simulink library "VLSGains"  (R2022b)
settings: Solver=VariableStepAuto  StartTime=0.0  StopTime=10.0  RelTol=1e-3
values from neighbouring files (symbols this model uses):
  VLSGainsConfig = struct('sample_rate_in_hertz', sample_rate_in_hertz,                              'frame_size', frame_size,                              'rgain_SILENT_GAIN', rgain_SILENT_GAIN,                              'granularity', internal_granularity,                              'numGains', numGains)    [VLSGainsInit.m]
  VLSGainsTune = load(VLSGainsTuneFileName)    [VLSGainsInit.m]
undefined symbols (not defined in the file or in its folder): Row
libraries: TuneVar x36, TOP x18, FeaturePath x2
(part 2 of 2)

== matlab function VLSGains/VLS Gains Pax/Fade Tuning/Forward Downmix Threshold/Trivial Translation ==
  data: TOP output; ForwardDownmixThreshold input
  events: trigger input FUNCTION_CALL_EVENT
function TOP  = fcn(ForwardDownmixThreshold)
%#codegen
% Checks if the parameter satisfies dimensionality requirements
if(numel(ForwardDownmixThreshold.Value) ~= 1)
   TranslateError('The parameter ''medusa_forward_downmix_threshold'' must be single dimensional.'); 
end

% Checks if the parameter value follows bound requirements
if((ForwardDownmixThreshold.Value < 0) || (ForwardDownmixThreshold.Value > 1))
   TranslateError('The value of ''medusa_forward_downmix_threshold'' must be between 0 and 1.'); 
end

TOP = ForwardDownmixThreshold.Value;

end

== matlab function VLSGains/VLS Gains Pax/Fade Tuning/Foward Downmix Max/Trivial Translation ==
  data: TOP output; ForwardDownmixMax input
  events: trigger input FUNCTION_CALL_EVENT
function TOP  = fcn(ForwardDownmixMax)
%#codegen
% Checks if the parameter satisfies dimensionality requirements
if(numel(ForwardDownmixMax.Value) ~= 1)
   TranslateError('The parameter ''medusa_forward_downmix_max'' must be single dimensional.'); 
end

% Checks if the parameter value follows bound requirements
if((ForwardDownmixMax.Value < 0) || (ForwardDownmixMax.Value > 1))
   TranslateError('The value of ''medusa_forward_downmix_max'' must be between 0 and 1.'); 
end

TOP = ForwardDownmixMax.Value;

end

== matlab function VLSGains/VLS Gains Pax/Gain Computation/Fader Downmix/MATLAB Function ==
  data: forwardGain input; downmix output; forwardDownmixThreshold input; forwardDownmixMax input; backwardGain input; backwardDownmixThreshold input; backwardDownmixMax input
function downmix = fcn(forwardGain, forwardDownmixThreshold, forwardDownmixMax,...
    backwardGain, backwardDownmixThreshold, backwardDownmixMax)

if (forwardGain >= backwardGain)
    downmix = (1 - min(backwardGain, forwardDownmixThreshold) / max(forwardDownmixThreshold, single(eps)))...
        * forwardDownmixMax;
else
    downmix = (1 - min(forwardGain, backwardDownmixThreshold) / max(backwardDownmixThreshold, single(eps)))...
        * backwardDownmixMax;
end

== matlab function VLSGains/VLS Gains Pax/Gain Computation/Ramper/check sequence ==
  data: done output; VLSPax_currentGain data_store_memory; VLSPax_targetGain data_store_memory
  events: trigger input FUNCTION_CALL_EVENT
function done = GetCompletedSequence
% #codegen

    global VLSPax_currentGain;
    global VLSPax_targetGain;

    % Assume the work is complete until proven otherwise
    done = true;

    for i=1:numel(VLSPax_targetGain)
       if (VLSPax_targetGain(i) ~= VLSPax_currentGain(i))
           done = false; % just proved otherwise
           break;
       end
    end

end

== matlab function VLSGains/VLS Gains Pax/Gain Computation/Ramper/control ==
  data target_gains_linear settings: description=This vector signal must provide a linear target gain for every ramper.
  data: target_gains_linear input; rampRate input; rampTime input; configStruct parameter; VLSPax_Freeze data_store_memory; VLSPax_frameCount data_store_memory; VLSPax_rampCoeff data_store_memory; VLSPax_targetGain data_store_memory; VLSPax_currentGain data_store_memory
  events: trigger input FUNCTION_CALL_EVENT
function control(target_gains_linear, rampRate, rampTime, configStruct)
%#codegen

    global VLSPax_Freeze;
    global VLSPax_frameCount;
    global VLSPax_rampCoeff;
    global VLSPax_targetGain;
    global VLSPax_currentGain;  

    dim_rgain = size(VLSPax_currentGain);
    rgain_SILENT_GAIN_mat = (configStruct.rgain_SILENT_GAIN)*ones(dim_rgain);

    % Step 1: FREEZE the gain ramper so that we can perform calculations based
    % on the current gain value.
    VLSPax_Freeze(1) = true; % freeze the gain

    % Step 2: Nudge the gain values a bit if they are sitting at zero.
    % When this control set goes live, ensure that the current gain will move.
    % If current gain is zero, replace with a value very close to zero. What we
    % really want is a value which is on the edge of perception - not too small
    % or large. If the value is too small, we'll waste some of our ramp time
    % in perceived silence. If the value is too large, the audio will lurch
    % into perceptability at the start of the ramp.
    currentgain = max(VLSPax_currentGain, rgain_SILENT_GAIN_mat);
    targetGain  = max(target_gains_linear, rgain_SILENT_GAIN_mat);
    
    % Step 3a: If a ramp time in milliseconds is provided, ignore the ramp
    % rate in dB/sec (if also provided), otherwise calculate a new ramp time
    % that matches the slope.
    rampTime_ms = single(rampTime)*ones(dim_rgain);
    
    if(~rampTime)
        currentGain_db = 20*log10(currentgain);
        targetGain_db = 20*log10(targetGain);
        diff = abs(currentGain_db - targetGain_db);
        rampTime_ms = diff / single(rampRate) * 1000;
    end
    
    % Step 3b: QUANTIZE the desired ramp time to our FrameSize. Also retrieve 
    % the whole number of frames required to best match requested ramp time.
    % Ensure that at least one frame is used. The frame size will therefore
    % determine the steepest ramp (i.e. within one frame you can go anywhere).
    quantum_ms = 1000 * (configStruct.frame_size) / (configStruct.sample_rate_in_hertz);
    numFrames = rampTime_ms / quantum_ms;
    numFrames = max (1, round(numFrames));

    % In order to have the desired ramp time, the slope must vary dependent
    % on the gain differencebetween target and current value.
    % Ramper's coefficient is therefore calculated as follows:
    %
    %   TargetGain = CurrentGain *( RampCoef ^ (Fs*RampTime_ms/1000) )
    %
    % therefore...
    %
    %                     log(TargetGain/CurrentGain)
    %   log(RampCoef) = ------------------------------
    %                        Fs*(RampTime_ms/1000)
    %
    factor = log( targetGain ./ currentgain );
    RampCoef = exp(factor ./ numFrames);

    % Output control signals
    VLSPax_frameCount  = int32(numFrames);
    VLSPax_rampCoeff   = single(RampCoef);
    VLSPax_targetGain  = target_gains_linear;
    VLSPax_currentGain = currentgain;

    % unfreeze the gain
    VLSPax_Freeze(1) = false;

end

== matlab function VLSGains/VLS Gains Pax/Gain Computation/Ramper/process ==
  data: VLSPax_Freeze data_store_memory; VLSPax_currentGain data_store_memory; VLSPax_targetGain data_store_memory; VLSPax_frameCount data_store_memory; VLSPax_rampCoeff data_store_memory
function process
%#codegen

    global VLSPax_Freeze;
    global VLSPax_currentGain;
    global VLSPax_targetGain;
    global VLSPax_frameCount;
    global VLSPax_rampCoeff;
    
    for i = 1:numel(VLSPax_currentGain)
        if (VLSPax_Freeze(1) == false)
            if (VLSPax_frameCount(i) == 0)
                % The ramp is finished. Stop ramping and SNAP to the target
                VLSPax_currentGain(i) = VLSPax_targetGain(i);
            else
                % The ramp is *NOT* frozen or done: gain is moving
                VLSPax_currentGain(i) = VLSPax_currentGain(i)*VLSPax_rampCoeff(i);
                VLSPax_frameCount(i) = VLSPax_frameCount(i) - 1;
            end
        end
    end
    
end

== matlab function VLSGains/VLS Gains Drv/Gain Computation/Fader Downmix/MATLAB Function ==
  data: forwardGain input; downmix output; forwardDownmixThreshold input; forwardDownmixMax input; backwardGain input; backwardDownmixThreshold input; backwardDownmixMax input
function downmix = fcn(forwardGain, forwardDownmixThreshold, forwardDownmixMax,...
    backwardGain, backwardDownmixThreshold, backwardDownmixMax)

if (forwardGain >= backwardGain)
    downmix = (1 - min(backwardGain, forwardDownmixThreshold) / max(forwardDownmixThreshold, single(eps)))...
        * forwardDownmixMax;
else
    downmix = (1 - min(forwardGain, backwardDownmixThreshold) / max(backwardDownmixThreshold, single(eps)))...
        * backwardDownmixMax;
end

== matlab function VLSGains/VLS Gains Drv/Gain Computation/Surround Level Control/Initialization and RMDL ==
  data: minGain input; detentGain input; maxGain input; interpolation_method input; surr_level input; configStruct parameter; VLSDrv_currentGain data_store_memory; VLSDrv_targetGain data_store_memory; VLSDrv_frameCount data_store_memory; VLSDrv_SLCGain data_store_memory
  events: trigger input FUNCTION_CALL_EVENT
function generate_gain(minGain, detentGain, maxGain, interpolation_method, surr_level, configStruct)
% #codegen
    global VLSDrv_currentGain;
    global VLSDrv_targetGain;
    global VLSDrv_SLCGain;
    global VLSDrv_frameCount;

    % Computing the 'surround' part of mixing gains depending on the surround
    % level index; The other part of mixing gain comes from 'fade downmix'
    gain = MedusaPremixGainComputation(minGain, detentGain, maxGain, interpolation_method, surr_level, configStruct);

    % Ramping doesn't take place during RMDL and cold start. Hence, gains
    % are directly pushed to mixing matrix
    VLSDrv_currentGain = gain;
    VLSDrv_targetGain = gain;
    VLSDrv_SLCGain = gain;
    
    % Resetting the frame count to zero to avoid unintentional ramping
    VLSDrv_frameCount = zeros(size(VLSDrv_currentGain), 'int32');
end

== matlab function VLSGains/VLS Gains Pax/Gain Computation/Surround Level Control/Initialization and RMDL ==
  data: minGain input; detentGain input; maxGain input; interpolation_method input; surr_level input; configStruct parameter; VLSPax_currentGain data_store_memory; VLSPax_targetGain data_store_memory; VLSPax_frameCount data_store_memory; VLSPax_SLCGain data_store_memory
  events: trigger input FUNCTION_CALL_EVENT
function generate_gain(minGain, detentGain, maxGain, interpolation_method, surr_level, configStruct)
% #codegen
    global VLSPax_currentGain;
    global VLSPax_targetGain;
    global VLSPax_SLCGain;
    global VLSPax_frameCount;

    % Computing the 'surround' part of mixing gains depending on the surround
    % level index; The other part of mixing gain comes from 'fade downmix'
    gain = MedusaPremixGainComputation(minGain, detentGain, maxGain, interpolation_method, surr_level, configStruct);

    % Ramping doesn't take place during RMDL and cold start. Hence, gains
    % are directly pushed to mixing matrix
    VLSPax_currentGain = gain;
    VLSPax_targetGain = gain;
    VLSPax_SLCGain = gain;
    
    % Resetting the frame count to zero to avoid unintentional ramping
    VLSPax_frameCount = zeros(size(VLSPax_currentGain), 'int32');
end

== matlab function VLSGains/VLS Gains Pax/Gain Computation/Surround Level Control/Target Gain Computation ==
  data: minGain input; detentGain input; maxGain input; interpolation_method input; surr_level input; configStruct parameter; VLSPax_SLCGain data_store_memory
  events: trigger input FUNCTION_CALL_EVENT
function generate_gain(minGain, detentGain, maxGain, interpolation_method, surr_level, configStruct)
% #codegen
    global VLSPax_SLCGain;

    % Computing the 'surround' part of mixing gains depending on the surround
    % level index; The other part of mixing gain comes from 'fade downmix'
    targetGain = MedusaPremixGainComputation(minGain, detentGain, maxGain, interpolation_method, surr_level, configStruct);
    
    VLSPax_SLCGain = targetGain;
end

== matlab function VLSGains/VLS Gains Pax/Generate Ramp Trigger/MATLAB Function ==
  data: SLC_On input; Fade_On input; rampOn output
  events: ramp output FUNCTION_CALL_EVENT
function rampOn = triggerRamp(SLC_On, Fade_On)
%#codegen
rampOn = 0;         % DEBUG parameter

% Trigger ramping if SLC OR Fade is triggered
if(SLC_On || Fade_On)
    rampOn = 1;
    ramp();
end

end

== matlab function VLSGains/VLS Gains Pax/SLC Tuning/Detent Level/Trivial Translation ==
  data: TOP output; detentGain input; configStruct parameter
  events: trigger input FUNCTION_CALL_EVENT
function TOP  = fcn(detentGain, configStruct)
%#codegen

% Checks if the parameter satisfies dimensionality requirements
if(detentGain.Size(1) ~= configStruct.numGains)
    TranslateError('The parameter ''VLS_gains_detent'' must be a %d element vector.', configStruct.numGains);
end

% Checks if the parameter values follow bound requirements
checkValues = (detentGain.Value < 0);    
if(sum(sum(checkValues)))       % Results in 0 if all values in the matrix respect the bound requirements
    TranslateError('The weights in ''VLS_gains_detent'' must be greater than or equal to 0.');
end

TOP = detentGain.Value;

end

== matlab function VLSGains/VLS Gains Pax/SLC Tuning/Interpolation Method/Trivial Translation ==
  data: TOP output; interpolationMethod input
  events: trigger input FUNCTION_CALL_EVENT
function TOP  = fcn(interpolationMethod)
%#codegen
% Checks if the parameter satisfies dimensionality requirements
if(numel(interpolationMethod.Value) ~= 1)
   TranslateError('The parameter ''medusa_surround_db_interpolation'' must be single dimensional.'); 
end

% Checks if the parameter value follows bound requirements
if((interpolationMethod.Value ~= 0) && (interpolationMethod.Value ~= 1))
   TranslateError('The value of ''medusa_surround_db_interpolation'' must be either 0 (for linear interpolation) or 1 (for dB-linear interpolation).'); 
end

TOP = interpolationMethod.Value;

end

== matlab function VLSGains/VLS Gains Pax/SLC Tuning/Max Level/Trivial Translation ==
  data: TOP output; maxGain input; configStruct parameter
  events: trigger input FUNCTION_CALL_EVENT
function TOP  = fcn(maxGain, configStruct)
%#codegen

% Checks if the parameter satisfies dimensionality requirements
if(maxGain.Size(1) ~= configStruct.numGains)
    TranslateError('The parameter ''VLS_gains_max'' must be a %d element vector.', configStruct.numGains);
end

% Checks if the parameter values follow bound requirements
checkValues = (maxGain.Value < 0);
if(sum(sum(checkValues)))          % Results in 0 if all values in the matrix respect the bound requirements
    TranslateError('The weights in ''VLS_gains_max'' must be greater than or equal to 0.');
end

TOP = maxGain.Value;

end

== matlab function VLSGains/VLS Gains Pax/SLC Tuning/Min Level/Trivial Translation ==
  data: TOP output; minGain input; configStruct parameter
  events: trigger input FUNCTION_CALL_EVENT
function TOP  = fcn(minGain, configStruct)
%#codegen

% Checks if the parameter satisfies dimensionality requirements
if(minGain.Size(1) ~= configStruct.numGains)
    TranslateError('The parameter ''VLS_gains_min'' must be a %d element vector.', configStruct.numGains);
end

% Checks if the parameter values follow bound requirements
checkValues = (minGain.Value < 0);
if(sum(sum(checkValues)))          % Results in 0 if all values in the matrix respect the bound requirements
    TranslateError('The weights in ''VLS_gains_min'' must be greater than or equal to 0.');
end

TOP = minGain.Value;

end

== matlab function VLSGains/VLS Gains Drv/Gain Computation/Surround Level Control/Target Gain Computation ==
  data: minGain input; detentGain input; maxGain input; interpolation_method input; surr_level input; configStruct parameter; VLSDrv_SLCGain data_store_memory
  events: trigger input FUNCTION_CALL_EVENT
function generate_gain(minGain, detentGain, maxGain, interpolation_method, surr_level, configStruct)
% #codegen
    global VLSDrv_SLCGain;

    % Computing the 'surround' part of mixing gains depending on the surround
    % level index; The other part of mixing gain comes from 'fade downmix'
    targetGain = MedusaPremixGainComputation(minGain, detentGain, maxGain, interpolation_method, surr_level, configStruct);
    
    VLSDrv_SLCGain = targetGain;
end

== matlab function VLSGains/VLS Gains Drv/SLC Tuning/Detent Level/Trivial Translation ==
  data: TOP output; detentGain input; configStruct parameter
  events: trigger input FUNCTION_CALL_EVENT
function TOP  = fcn(detentGain, configStruct)
%#codegen

% Checks if the parameter satisfies dimensionality requirements
if(detentGain.Size(1) ~= configStruct.numGains)
    TranslateError('The parameter ''VLS_gains_detent'' must be a %d element vector.', configStruct.numGains);
end

% Checks if the parameter values follow bound requirements
checkValues = (detentGain.Value < 0);    
if(sum(sum(checkValues)))       % Results in 0 if all values in the matrix respect the bound requirements
    TranslateError('The weights in ''VLS_gains_detent'' must be greater than or equal to 0.');
end

TOP = detentGain.Value;

end

== matlab function VLSGains/VLS Gains Drv/SLC Tuning/Interpolation Method/Trivial Translation ==
  data: TOP output; interpolationMethod input
  events: trigger input FUNCTION_CALL_EVENT
function TOP  = fcn(interpolationMethod)
%#codegen
% Checks if the parameter satisfies dimensionality requirements
if(numel(interpolationMethod.Value) ~= 1)
   TranslateError('The parameter ''medusa_surround_db_interpolation'' must be single dimensional.'); 
end

% Checks if the parameter value follows bound requirements
if((interpolationMethod.Value ~= 0) && (interpolationMethod.Value ~= 1))
   TranslateError('The value of ''medusa_surround_db_interpolation'' must be either 0 (for linear interpolation) or 1 (for dB-linear interpolation).'); 
end

TOP = interpolationMethod.Value;

end

== matlab function VLSGains/VLS Gains Drv/SLC Tuning/Max Level/Trivial Translation ==
  data: TOP output; maxGain input; configStruct parameter
  events: trigger input FUNCTION_CALL_EVENT
function TOP  = fcn(maxGain, configStruct)
%#codegen

% Checks if the parameter satisfies dimensionality requirements
if(maxGain.Size(1) ~= configStruct.numGains)
    TranslateError('The parameter ''VLS_gains_max'' must be a %d element vector.', configStruct.numGains);
end

% Checks if the parameter values follow bound requirements
checkValues = (maxGain.Value < 0);
if(sum(sum(checkValues)))          % Results in 0 if all values in the matrix respect the bound requirements
    TranslateError('The weights in ''VLS_gains_max'' must be greater than or equal to 0.');
end

TOP = maxGain.Value;

end

== matlab function VLSGains/VLS Gains Drv/SLC Tuning/Min Level/Trivial Translation ==
  data: TOP output; minGain input; configStruct parameter
  events: trigger input FUNCTION_CALL_EVENT
function TOP  = fcn(minGain, configStruct)
%#codegen

% Checks if the parameter satisfies dimensionality requirements
if(minGain.Size(1) ~= configStruct.numGains)
    TranslateError('The parameter ''VLS_gains_min'' must be a %d element vector.', configStruct.numGains);
end

% Checks if the parameter values follow bound requirements
checkValues = (minGain.Value < 0);
if(sum(sum(checkValues)))          % Results in 0 if all values in the matrix respect the bound requirements
    TranslateError('The weights in ''VLS_gains_min'' must be greater than or equal to 0.');
end

TOP = minGain.Value;

end

== matlab function VLSGains/VLS Gains Drv/Gain Computation/Ramper/check sequence ==
  data: done output; VLSDrv_currentGain data_store_memory; VLSDrv_targetGain data_store_memory
  events: trigger input FUNCTION_CALL_EVENT
function done = GetCompletedSequence
% #codegen

    global VLSDrv_currentGain;
    global VLSDrv_targetGain;

    % Assume the work is complete until proven otherwise
    done = true;

    for i=1:numel(VLSDrv_targetGain)
       if (VLSDrv_targetGain(i) ~= VLSDrv_currentGain(i))
           done = false; % just proved otherwise
           break;
       end
    end

end

== matlab function VLSGains/VLS Gains Drv/Gain Computation/Ramper/control ==
  data target_gains_linear settings: description=This vector signal must provide a linear target gain for every ramper.
  data: target_gains_linear input; rampRate input; rampTime input; configStruct parameter; VLSDrv_Freeze data_store_memory; VLSDrv_frameCount data_store_memory; VLSDrv_rampCoeff data_store_memory; VLSDrv_targetGain data_store_memory; VLSDrv_currentGain data_store_memory
  events: trigger input FUNCTION_CALL_EVENT
function control(target_gains_linear, rampRate, rampTime, configStruct)
%#codegen

    global VLSDrv_Freeze;
    global VLSDrv_frameCount;
    global VLSDrv_rampCoeff;
    global VLSDrv_targetGain;
    global VLSDrv_currentGain;  

    dim_rgain = size(VLSDrv_currentGain);
    rgain_SILENT_GAIN_mat = (configStruct.rgain_SILENT_GAIN)*ones(dim_rgain);

    % Step 1: FREEZE the gain ramper so that we can perform calculations based
    % on the current gain value.
    VLSDrv_Freeze(1) = true; % freeze the gain

    % Step 2: Nudge the gain values a bit if they are sitting at zero.
    % When this control set goes live, ensure that the current gain will move.
    % If current gain is zero, replace with a value very close to zero. What we
    % really want is a value which is on the edge of perception - not too small
    % or large. If the value is too small, we'll waste some of our ramp time
    % in perceived silence. If the value is too large, the audio will lurch
    % into perceptability at the start of the ramp.
    currentgain = max(VLSDrv_currentGain, rgain_SILENT_GAIN_mat);
    targetGain  = max(target_gains_linear, rgain_SILENT_GAIN_mat);
    
    % Step 3a: If a ramp time in milliseconds is provided, ignore the ramp
    % rate in dB/sec (if also provided), otherwise calculate a new ramp time
    % that matches the slope.
    rampTime_ms = single(rampTime)*ones(dim_rgain);
    
    if(~rampTime)
        currentGain_db = 20*log10(currentgain);
        targetGain_db = 20*log10(targetGain);
        diff = abs(currentGain_db - targetGain_db);
        rampTime_ms = diff / single(rampRate) * 1000;
    end
    
    % Step 3b: QUANTIZE the desired ramp time to our FrameSize. Also retrieve 
    % the whole number of frames required to best match requested ramp time.
    % Ensure that at least one frame is used. The frame size will therefore
    % determine the steepest ramp (i.e. within one frame you can go anywhere).
    quantum_ms = 1000 * (configStruct.frame_size) / (configStruct.sample_rate_in_hertz);
    numFrames = rampTime_ms / quantum_ms;
    numFrames = max (1, round(numFrames));

    % In order to have the desired ramp time, the slope must vary dependent
    % on the gain differencebetween target and current value.
    % Ramper's coefficient is therefore calculated as follows:
    %
    %   TargetGain = CurrentGain *( RampCoef ^ (Fs*RampTime_ms/1000) )
    %
    % therefore...
    %
    %                     log(TargetGain/CurrentGain)
    %   log(RampCoef) = ------------------------------
    %                        Fs*(RampTime_ms/1000)
    %
    factor = log( targetGain ./ currentgain );
    RampCoef = exp(factor ./ numFrames);

    % Output control signals
    VLSDrv_frameCount  = int32(numFrames);
    VLSDrv_rampCoeff   = single(RampCoef);
    VLSDrv_targetGain  = target_gains_linear;
    VLSDrv_currentGain = currentgain;

    % unfreeze the gain
    VLSDrv_Freeze(1) = false;

end

== matlab function VLSGains/VLS Gains Drv/Gain Computation/Ramper/process ==
  data: VLSDrv_Freeze data_store_memory; VLSDrv_currentGain data_store_memory; VLSDrv_targetGain data_store_memory; VLSDrv_frameCount data_store_memory; VLSDrv_rampCoeff data_store_memory
function process
%#codegen

    global VLSDrv_Freeze;
    global VLSDrv_currentGain;
    global VLSDrv_targetGain;
    global VLSDrv_frameCount;
    global VLSDrv_rampCoeff;
    
    for i = 1:numel(VLSDrv_currentGain)
        if (VLSDrv_Freeze(1) == false)
            if (VLSDrv_frameCount(i) == 0)
                % The ramp is finished. Stop ramping and SNAP to the target
                VLSDrv_currentGain(i) = VLSDrv_targetGain(i);
            else
                % The ramp is *NOT* frozen or done: gain is moving
                VLSDrv_currentGain(i) = VLSDrv_currentGain(i)*VLSDrv_rampCoeff(i);
                VLSDrv_frameCount(i) = VLSDrv_frameCount(i) - 1;
            end
        end
    end
    
end

== matlab function VLSGains/VLS Gains Drv/Generate Ramp Trigger/MATLAB Function ==
  data: SLC_On input; Fade_On input; rampOn output
  events: ramp output FUNCTION_CALL_EVENT
function rampOn = triggerRamp(SLC_On, Fade_On)
%#codegen
rampOn = 0;         % DEBUG parameter

% Trigger ramping if SLC OR Fade is triggered
if(SLC_On || Fade_On)
    rampOn = 1;
    ramp();
end

end

== matlab function VLSGains/VLS Gains Drv/Fade Inputs/Fade_Trigger_Generation ==
  data: gainDifference input; fadeOn output
  events: fadeTrigger output FUNCTION_CALL_EVENT
function fadeOn = Fade_Trigger(gainDifference)
% #codegen
    fadeOn = false;
    
    % Generates function call triggers when incoming fade gain values change
    if(gainDifference > 0)
        fadeTrigger();
        fadeOn = true;      % Indicates that fade is triggered
    end
end

== matlab function VLSGains/VLS Gains Drv/Fade Tuning/Backward Downmix Max/Trivial Translation ==
  data: TOP output; BackwardDownmixMax input
  events: trigger input FUNCTION_CALL_EVENT
function TOP  = fcn(BackwardDownmixMax)
%#codegen
% Checks if the parameter satisfies dimensionality requirements
if(numel(BackwardDownmixMax.Value) ~= 1)
   TranslateError('The parameter ''medusa_backward_downmix_max'' must be single dimensional.'); 
end

% Checks if the parameter value follows bound requirements
if((BackwardDownmixMax.Value < 0) || (BackwardDownmixMax.Value > 1))
   TranslateError('The value of ''medusa_backward_downmix_max'' must be between 0 and 1.'); 
end

TOP = BackwardDownmixMax.Value;

end

== matlab function VLSGains/VLS Gains Pax/Fade Inputs/Fade_Trigger_Generation ==
  data: gainDifference input; fadeOn output
  events: fadeTrigger output FUNCTION_CALL_EVENT
function fadeOn = Fade_Trigger(gainDifference)
% #codegen
    fadeOn = false;
    
    % Generates function call triggers when incoming fade gain values change
    if(gainDifference > 0)
        fadeTrigger();
        fadeOn = true;      % Indicates that fade is triggered
    end
end

== matlab function VLSGains/VLS Gains Pax/Fade Tuning/Backward Downmix Max/Trivial Translation ==
  data: TOP output; BackwardDownmixMax input
  events: trigger input FUNCTION_CALL_EVENT
function TOP  = fcn(BackwardDownmixMax)
%#codegen
% Checks if the parameter satisfies dimensionality requirements
if(numel(BackwardDownmixMax.Value) ~= 1)
   TranslateError('The parameter ''medusa_backward_downmix_max'' must be single dimensional.'); 
end

% Checks if the parameter value follows bound requirements
if((BackwardDownmixMax.Value < 0) || (BackwardDownmixMax.Value > 1))
   TranslateError('The value of ''medusa_backward_downmix_max'' must be between 0 and 1.'); 
end

TOP = BackwardDownmixMax.Value;

end

== matlab function VLSGains/VLS Gains Drv/Fade Tuning/Backward Downmix Threshold/Trivial Translation ==
  data: TOP output; BackwardDownmixThreshold input
  events: trigger input FUNCTION_CALL_EVENT
function TOP  = fcn(BackwardDownmixThreshold)
%#codegen
% Checks if the parameter satisfies dimensionality requirements
if(numel(BackwardDownmixThreshold.Value) ~= 1)
   TranslateError('The parameter ''medusa_backward_downmix_threshold'' must be single dimensional.'); 
end

% Checks if the parameter value follows bound requirements
if((BackwardDownmixThreshold.Value < 0) || (BackwardDownmixThreshold.Value > 1))
   TranslateError('The value of ''medusa_backward_downmix_threshold'' must be between 0 and 1.'); 
end

TOP = BackwardDownmixThreshold.Value;

end
